simulink model "r_128w_8k_1a_16x_r431"  (R2012b)
settings: Solver=FixedStepDiscrete  SolverMode=SingleTasking  StartTime=0.0  StopTime=5000  RelTol=1e-3
undefined symbols (not defined in the file): Down, pfb_coeff_gen_calc, Up
libraries: xbsIndex_r4 x9410, casper_library_misc x257, casper_library_delays x92, xps_library x57, simulink x16, dspsigops x12, casper_library_flow_control x8, xbsReplacements_r4 x4, casper_library_multipliers x4, casper_library_scopes x2, casper_library_ffts_twiddle x2
(part 70 of 125)

== system r_128w_8k_1a_16x_r431/fft_wideband_real1/fft_direct/butterfly2_0/twiddle_general_dsp48e/coeff_gen ==
  rst : Inport
  Counter : xbsIndex_r4/Counter  cnt_type=Free Running  cnt_to=Inf  operation=Up  start_count=0  cnt_by_val=1  arith_type=Unsigned  n_bits=12  bin_pt=0  load_pin=off  rst=on  en=off  explicit_period=on  period=1  dbl_ovrd=off  use_behavioral_HDL=off  implementation=Fabric  block_type=counter
  ROM : xbsIndex_r4/ROM  depth=4096  initVector="[1                                      1                                      1                                      1                                      1                                      1                                      1                                      1                                      1                                      1                                      1                     0.9999847412109375                     0.9999847412109375                     0.9999847412109375                     0.9999847412109375                     0.9999847412109375                     0.9999847412109375                     0.9999847412109375                      0.999969482421875                      0.999969482421875                      0.999969482421875                      0.999969482421875                      0.999969482421875                     0.9999542236328125                     0.9999542236328125                     0.9999542236328125                     0.9999542236328125                       0.99993896484375                       0.99993896484375                       0.99993896484375                       0.99993896484375                     0.9999237060546875                     0.9999237060546875                     0.9999237060546875                      0.999908447265625                      0.999908447265625                      0.999908447265625                     0.9998931884765625                     0.9998931884765625                     0.9998931884765625                        0.9998779296875                        0.9998779296875                     0.9998626708984375                     0.9998626708984375                     0.9998626708984375                      0.999847412109375                      0.999847412109375                     0.9998321533203125                     0.9998321533203125                       0.99981689453125                       0.99981689453125                     0.9998016357421875                     0.9998016357421875                      0.999786376953125                      0.999786376953125                     0.9997711181640625                     0.9997711181640625                         0.999755859375                         0.999755859375                     0.9997406005859375                     0.9997406005859375                      0.999725341796875                     0.9997100830078125                     0.9997100830078125                       0.99969482421875                       0.99969482421875                     0.9996795654296875                      0.999664306640625                      0.999664306640625                     0.9996490478515625                        0.9996337890625                        0.9996337890625                     0.9996185302734375                      0.999603271484375                      0.999603271484375                     0.9995880126953125                       0.99957275390625                     0.9995574951171875                     0.9995574951171875                      0.999542236328125                     0.9995269775390625                          0.99951171875                          0.99951171875                     0.9994964599609375                      0.999481201171875                     0.9994659423828125                       0.99945068359375                       0.99945068359375                     0.9994354248046875                      0.999420166015625                     0.9994049072265625                        0.9993896484375                     0.9993743896484375                      0.999359130859375                     0.9993438720703125                     0.9993438720703125                       0.99932861328125                     0.9993133544921875                      0.999298095703125                     0.9992828369140625                         0.999267578125                     0.9992523193359375                      0.999237060546875 ...(+155708 chars)]"  distributed_mem=Block RAM  rst=off  init_reg=0  en=off  latency=2  gui_display_data_type=Fixed-point  arith_type="Signed  (2's comp)"  n_bits=18  bin_pt=16  preci_type=Single  exp_width=8  frac_width=24  dbl_ovrd=off  optimize=Area  use_rpm=on  block_type=sprom
  ROM1 : xbsIndex_r4/ROM  depth=4096  initVector="[0                    -0.0003814697265625                     -0.000762939453125                    -0.0011444091796875                    -0.0015411376953125                     -0.001922607421875                    -0.0023040771484375                        -0.002685546875                    -0.0030670166015625                     -0.003448486328125                    -0.0038299560546875                      -0.00421142578125                     -0.004608154296875                    -0.0049896240234375                         -0.00537109375                    -0.0057525634765625                     -0.006134033203125                    -0.0065155029296875                      -0.00689697265625                     -0.007293701171875                    -0.0076751708984375                        -0.008056640625                    -0.0084381103515625                     -0.008819580078125                    -0.0092010498046875                      -0.00958251953125                    -0.0099639892578125                    -0.0103607177734375                          -0.0107421875                    -0.0111236572265625                     -0.011505126953125                    -0.0118865966796875                      -0.01226806640625                    -0.0126495361328125                     -0.013031005859375                        -0.013427734375                    -0.0138092041015625                     -0.014190673828125                    -0.0145721435546875                      -0.01495361328125                    -0.0153350830078125                     -0.015716552734375                         -0.01611328125                    -0.0164947509765625                     -0.016876220703125                    -0.0172576904296875                      -0.01763916015625                    -0.0180206298828125                     -0.018402099609375                    -0.0187835693359375                    -0.0191802978515625                     -0.019561767578125                    -0.0199432373046875                      -0.02032470703125                    -0.0207061767578125                     -0.021087646484375                    -0.0214691162109375                       -0.0218505859375                     -0.022247314453125                    -0.0226287841796875                      -0.02301025390625                    -0.0233917236328125                     -0.023773193359375                    -0.0241546630859375                       -0.0245361328125                    -0.0249176025390625                    -0.0253143310546875                      -0.02569580078125                    -0.0260772705078125                     -0.026458740234375                    -0.0268402099609375                       -0.0272216796875                    -0.0276031494140625                     -0.027984619140625                      -0.02838134765625                    -0.0287628173828125                     -0.029144287109375                    -0.0295257568359375                       -0.0299072265625                    -0.0302886962890625                     -0.030670166015625                    -0.0310516357421875                    -0.0314483642578125                     -0.031829833984375                    -0.0322113037109375                       -0.0325927734375                    -0.0329742431640625                     -0.033355712890625                    -0.0337371826171875                      -0.03411865234375                    -0.0345001220703125                    -0.0348968505859375                       -0.0352783203125                    -0.0356597900390625                     -0.036041259765625                    -0.0364227294921875                      -0.03680419921875                    -0.0371856689453125                     -0.037567138671875                       -0.0379638671875                    -0.0383453369140625                     -0.038726806640625                    -0.0391082763671875 ...(+155708 chars)]"  distributed_mem=Block RAM  rst=off  init_reg=0  en=off  latency=2  gui_display_data_type=Fixed-point  arith_type="Signed  (2's comp)"  n_bits=18  bin_pt=16  preci_type=Single  exp_width=8  frac_width=24  dbl_ovrd=off  optimize=Area  use_rpm=on  block_type=sprom
  Slice : xbsIndex_r4/Slice  nbits=12  boolean_output=off  mode=Upper Bit Location + Width  bit1=0  base1=MSB of Input  bit0=0  base0=LSB of Input  dbl_ovrd=off  block_type=slice
  ri_to_c : casper_library_misc/ri_to_c
  w : Outport
  wires:
  ri_to_c/1 -> w/1
  rst/1 -> Counter/1
  Counter/1 -> Slice/1
  Slice/1 -> ROM/1, ROM1/1
  ROM/1 -> ri_to_c/1
  ROM1/1 -> ri_to_c/2
